simulink model "TEST_yuyao_all_BASIC_v2"  (R2023a)
settings: Solver=FixedStepDiscrete  StartTime=0.0  StopTime=inf  FixedStep=0.001  RelTol=1e-3  EnableMultiTasking=on
undefined symbols (not defined in the file or in its folder): IO397
libraries: slrealtimeseriallib x3, speedgoatlib_fpga_dio x2, speedgoatlib_fpga_analog_io x1, speedgoatlib_fpga x1
settings Model: Creator=Kalpana  LastModifiedBy=ysun
settings SolverCC: ConcurrentTasks=on  AlgebraicLoopSolver=TrustRegion  PositivePriorityOrder=on  InsertRTBMode=Never (minimum delay)
settings DataIOCC: SaveFormat=Array  SaveState=on  SignalLoggingName=logsOut
settings OptimizationCC: BlockReduction=off  BooleanDataType=off  OptimizeBlockIOStorage=off  BufferReuse=off  ReuseModelBlockBuffer=off  GlobalBufferReuse=off  ExpressionFolding=off  LocalBlockOutputs=off  InitFltsAndDblsToZero=on  OptimizeDataStoreBuffers=off  BusAssignmentInplaceUpdate=off
settings DebuggingCC: SaveWithParameterizedLinksMsg=none  UnderspecifiedInitializationDetection=Classic  MergeDetectMultiDrivingBlocksExec=none  CheckExecutionContextPreStartOutputMsg=on  SignalResolutionControl=TryResolveAllWithWarning  TasksWithSamePriorityMsg=none  UnconnectedInputMsg=warning  UnconnectedOutputMsg=warning  UnconnectedLineMsg=warning  SFUnexpectedBacktrackingDiag=warning  SFNoUnconditionalDefaultTransitionDiag=warning  SFExecutionAtInitializationDiag=none  ArithmeticOperatorsInVariantConditions=warning
settings HardwareCC: ProdBitPerLong=64  ProdLongLongMode=on  ProdHWDeviceType=Intel->x86-64 (Linux 64)
settings ModelReferenceCC: EnableRefExpFcnMdlSchedulingChecks=on  PropagateSignalLabelsOutOfModel=off
settings SFSimCC: SimUseLocalCustomCode=off  SimTargetLang=C++
settings RTWCC: Description=Simulink Real-Time  SystemTargetFile=slrealtime.tlc  TemplateMakefile=slrealtime_default_tmf  RTWUseLocalCustomCode=off  Toolchain=Simulink Real-Time Toolchain  BuildConfiguration=Faster Runs  CodeExecutionProfiling=on  TargetLang=C++  DLArmComputeVersion=19.05
settings CodeAppCC: StateflowObjectComments=on
settings SimulinkRealTimeTargetCC: MATLABClassNameForMDSCustomization=Simulink.SoftwareTarget.GRTCustomization  UseGCCFastMath=on
settings ConfigComp: CovMetricSettings=dw  CovSaveCumulativeToWorkspaceVar=on  CovSaveSingleToWorkspaceVar=on  CovExternalEMLEnable=off  CovSFcnEnable=off

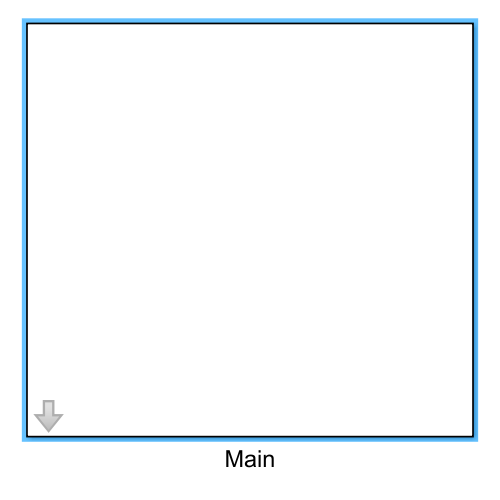
[thumbnail: Simulink's stored preview of the top-level diagram]
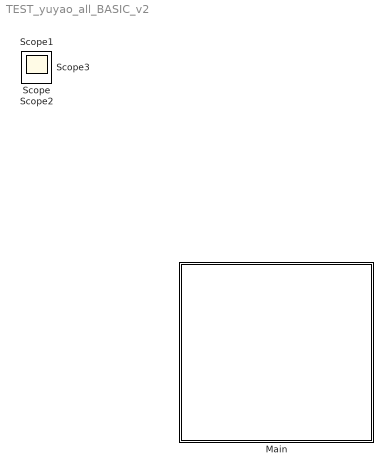
== system TEST_yuyao_all_BASIC_v2 ==
  Main : Subsystem  mask{iti_time=1, opp_time=500, deadtime=1000, water_time=1000, reaction_time=1000, target=10000}
      mask prompts: iti_time "inter trial interval duration (secs)"; opp_time "opportunity time (ms)"; deadtime "lick dead time (ms)"; water_time "water duration (ms)"; reaction_time "reaction_time(ms)"
      mask DialogControl win_parameters Prompt: Time Windows
  Scope{,1..3} (4 alike) : Scope

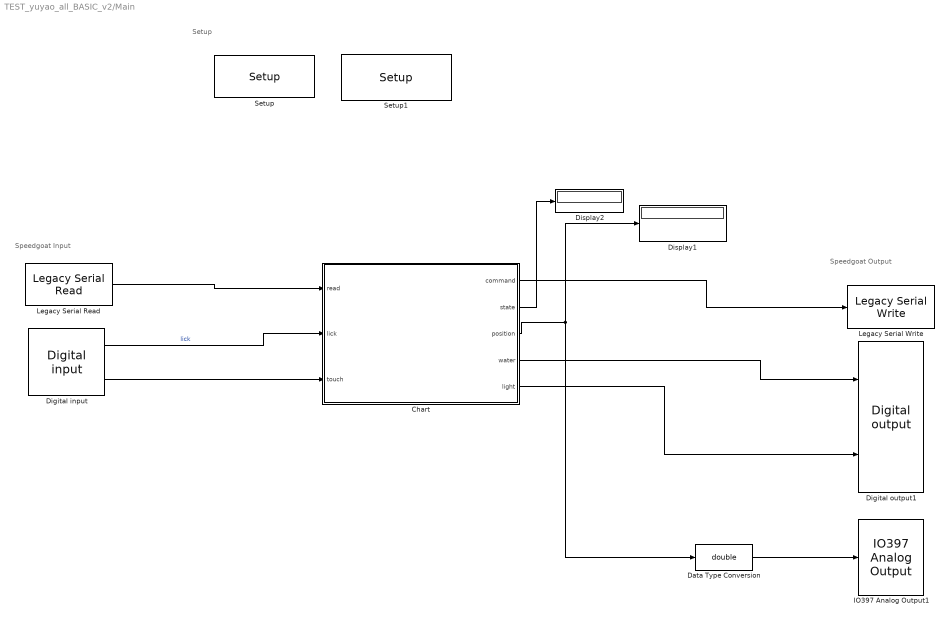
== system TEST_yuyao_all_BASIC_v2/Main ==
  note: Setup
  note: Speedgoat Input
  note: Speedgoat Output
  Chart : Stateflow chart  TreatAsAtomicUnit=on
      settings: PortSchema="{\"entries\":[{\"content\":{\"sides\":[{\"content\":{\"connectorIds\":[\"In1\",\"In2\",\"In3\"]},\"type\":\"ConnectorPlacement.EquallySpacedRectSide\",\"uuid\":\"c5c6425b-c61c-4cfd-8e89-a1433c662b1e\"},{\"content\":{\"connectorIds\":[\"Out1\",\"Out2\",\"Out3\",\"Out5\",\"Out4\"],\"side\":\"RIGHT\"},\"type\":\"ConnectorPlacement.EquallySpacedRectSide\",\"uuid\":\"e94e3558-7670-4901-8dc6-dcc10f25bbba\"},{\"content\":{\"side\":\"TOP\"},\"type\":\"ConnectorPlacement.EquallySpacedRectSide\",\"uuid\":\"e6d8a198-ffcd-48fe-900a-ac2ec65948b6\"}]},\"type\":\"ConnectorPlacement.EquallySpacedConnector\",\"uuid\":\"3d425b26-b95c-4585-983d-1dedea8cf8d0\"}],\"packageUris\":[\"http://schema.mathworks.com/mf0/Connector/R2020b\"],\"version\":\"1.0\"}"
  Data Type Conversion : DataTypeConversion  OutDataTypeStr=double  SaturateOnIntegerOverflow=off  RndMeth=Floor
  Digital input : speedgoatlib_fpga_dio/Digital input  id=1  chan=[1 5]  ts=0.01  pciSlot=-1  board=IO397-50k  vectorizeOutput=off
      settings: SourceProductName=Simulink Real-Time: Speedgoat I/O Blockset
  Digital output1 : speedgoatlib_fpga_dio/Digital output  id=1  chan=[2 6]  init=[0]  reset=[0]  vectorizeInput=off  ts=-1  pciSlot=-1  board=IO397-50k
      settings: SourceProductName=Simulink Real-Time: Speedgoat I/O Blockset
  Display1 : Display
  Display2 : Display
  IO397 Analog Output1 : speedgoatlib_fpga_analog_io/IO397 Analog Output  id=1  chan=[2]  initVal=0  resetVal=0  ts=0.01  pciSlot=-1  board=IO397-50k  span=+-5 V
      settings: SourceProductName=Simulink Real-Time: Speedgoat I/O Blockset
  Legacy Serial Read : slrealtimeseriallib/Mainboard/Legacy Serial Read  port=Legacy Serial Port 1  count=51  dtype=count+16 bit int  sampletime=.01
  Legacy Serial Write : slrealtimeseriallib/Mainboard/Legacy Serial Write  port=Legacy Serial Port 1  dtype=count+16 bit int  sampletime=.01
  Setup : slrealtimeseriallib/Mainboard/Setup  port=Legacy Serial Port 1  baud=115200  width=8  nstop=1  parity=None  ctsmode=off
  Setup1 : speedgoatlib_fpga/Setup/Setup  board=IO397-50k  id=1  device_id=1  frontIO=None  rearIO=None  bitstreamFile=speedgoat_IO397_50k_Comms.mat  rev=5.000000  timestamp_string=28/02/23 11:36:55  fpgaFreq=75 MHz  fpgaTick=13.33 ns  ProgSpiFlash=off  ProgBPIFlash=off  pciSlot=-1  PullRPort0=pull-up 3.3V  VioPort0=3.3V  PullRPort1=pull-up 3.3V  VioPort1=3.3V  PullRPort2=pull-up 3.3V  VioPort2=3.3V  PullRPort3=pull-up 3.3V  VioPort3=3.3V  PullRPort4=pull-up 3.3V  VioPort4=3.3V  PullRPort5=pull-up 3.3V  VioPort5=3.3V  PullRPort6=pull-up 3.3V  VioPort6=3.3V  diffLineTermination_rear1=on  diffLineTermination_rear2=on  diffLineTermination_rear3=on  diffLineTermination_rear4=on  diffLineTermination_rear5=on  diffLineTermination_rear6=on  diffLineTermination_rear7=on  diffLineTermination_rear8=on  PullRPort15=pull-up 3.3V  PullRPort31=pull-up 3.3V  PullRPort47=pull-up 3.3V  PullRPort63=pull-up 3.3V  diffLineTermination_1=on  diffLineTermination_2=on  diffLineTermination_3=on  diffLineTermination_4=on  diffLineTermination_5=on  diffLineTermination_6=on  diffLineTermination_7=on  diffLineTermination_8=on
      settings: SourceProductName=Simulink Real-Time: Speedgoat I/O Blockset
  wires:
  Data Type Conversion/1 -> IO397 Analog Output1/1
  Digital input/2 -> Chart/3(touch)
  Chart/5(water) -> Digital output1/1
  Legacy Serial Read/1 -> Chart/1(read)
  Chart/2(state) -> Display2/1
  Chart/1(command) -> Legacy Serial Write/1
  Chart/3(position) -> Data Type Conversion/1, Display1/1
  Chart/4(light) -> Digital output1/2
  Digital input/1 -> Chart/2(lick)  "lick"

== stateflow chart TEST_yuyao_all_BASIC_v2/Main/Chart ==
  state Motor
    entry:
    state = 0;
    during:
    on setenable_1: command =  int16([0x0014 0x0090 0x0002 0x0068 0x0004 0x0001 0x0040 0x0060 0x0000 0x0006 0x0000 0x0000 0x0000 0x0022 0x0099]);
    on setenable_2: command =  int16([0x0014 0x0090 0x0002 0x0068 0x0004 0x0001 0x0040 0x0060 0x0000 0x000F 0x0000 0x0000 0x0000 0x00B3 0x0007]);
    on clearerror_1: command =  int16([0x0014 0x0090 0x0002 0x0068 0x0004 0x0001 0x0003 0x0010 0x0000 0x0000 0x0000 0x0000 0x0000 0x00A1 0x0008]);
    on clearerror_2: command =  int16([0x0014 0x0090 0x0002 0x0068 0x0004 0x0001 0x0040 0x0060 0x0000 0x0000 0x0000 0x0000 0x0000 0x0082 0x002B]);
    on clearerror_3: command =  int16([0x0014 0x0090 0x0002 0x0068 0x0004 0x0001 0x0040 0x0060 0x0000 0x0080 0x0000 0x0000 0x0000 0x00D8 0x0010]);
    on getposition: command =  int16([0x0010 0x0090 0x0002 0x0060 0x0002 0x0001 0x0064 0x0060 0x0000 0x0029 0x005A 0x0000 0x0000 0x0000 0x0000 ]);
    on SetoperationMode: command = int16([0x0014 0x0090 0x0002 0x0068 0x0004 0x0001 0x0060 0x0060 0x0000 0x0001 0x0000 0x0000 0x0000 0x00DA 0x0067]);
    on getmovementstate: command = int16([0x0010 0x0090 0x0002 0x0060 0x0002 0x0001 0x0041 0x0060 0x0000 0x0022 0x00D1 0x0000 0x0000 0x0000 0x0000]);
    on Torque_mode: command = int16([0x0014 0x0090 0x0002 0x0068 0x0004 0x0001 0x0060 0x0060 0x0000 0x000A 0x0000 0x0000 0x0000 0x002B 0x0097]);
    on Torque: command = int16([0x0014 0x0090 0x0002 0x0068 0x0004 0x0001 0x0071 0x0060 0x0000 0x0030 0x00F8 0x00FF 0x00FF 0x00A9 0x00E8]);
    on setdisable:command = int16([0x0014 0x0090 0x0002 0x0068 0x0004 0x0001 0x0040 0x0060 0x0000 0x0000 0x0000 0x0000 0x0000 0x0082 0x002B]);
    on CSP_mode: command = int16([0x0014 0x0090 0x0002 0x0068 0x0004 0x0001 0x0060 0x0060 0x0000 0x0008 0x0000 0x0000 0x0000 0x004B 0x00F9]);
    on moveto0: command = int16([0x0014 0x0090 0x0002 0x0068 0x0004 0x0001 0x007A 0x0060 0x0000 0x0000 0x0000 0x0000 0x0000 0x0022 0x00FC]);
    state Getposition
      entry:
      getposition
      during:
      position = extractAndMerge(read);
      state State
        en:
        state = 2;
      state Pull
        en:
        state = 3;
      (default) -> State
      State -> Pull : [any(position >= target)]
    state ITI
    state ProgStart
      state SETENABLE_2
        entry:
        setenable_2
      state CLEARERROR
        entry:
        clearerror_1
      state SETENABLE
        entry:
        setenable_1
      state exit
        entry:
        state = 1;
      state CLEARERROR2
        entry:
        clearerror_2
      state CLEARERROR3
        entry:
        clearerror_3
      (default) -> Motor.ProgStart.SETENABLE
      Motor.ProgStart.SETENABLE_2 -> CLEARERROR : [after(10,msec)]
      Motor.ProgStart.SETENABLE -> Motor.ProgStart.SETENABLE_2 : [after(10,msec)]
      CLEARERROR -> CLEARERROR2 : [after(10,msec)]
      CLEARERROR2 -> CLEARERROR3 : [after(10,msec)]
      CLEARERROR3 -> exit : [after(10,msec)]
    state wait
    state lightOFF
      entry:
      light=0;
    state LightON
      entry:
      light=1;
    state WaterON
      entry:
      water = 1;
      ex:
      state = 6;
    state WaterOFF
      entry:
      water = 0;
    state Lickingtime
    state Getposition2
      entry:
      getposition
      during:
      position = extractAndMerge(read);
      state Position1
      state Position2
        en:
        state = 8;
      state Position3
        en:
        state =9;
      (default) -> Position1
      Position1 -> Position2 [order 1] : [any(position <= 500)]
      Position1 -> Position3 [order 4] : [any(position < -500)]
      Position1 -> Position3 [order 3] : [any(position > 500)]
      Position1 -> Position2 [order 2] : [any(position >= -500)]
    state ToMidpoint
      state SETENABLE_2
        entry:
        setenable_2
      state SETENABLE
        entry:
        setenable_1
      state CSP
        entry:
        CSP_mode
      state Torque
        en:
        Torque
      state MOVE
        entry:
        moveto0
      state MOVE1
        entry:
        state = 7;
      (default) -> Motor.ToMidpoint.SETENABLE
      Motor.ToMidpoint.SETENABLE -> Motor.ToMidpoint.SETENABLE_2 : [after(10,msec)]
      Motor.ToMidpoint.SETENABLE_2 -> CSP : [after(10,msec)]
      CSP -> Torque : [after(10,msec)]
      Torque -> MOVE : [after(10,msec)]
      MOVE -> MOVE1 : [after(10,msec)]
    ProgStart -> ITI : [state == 1]
    ITI -> Getposition : [after(iti_time,sec)]
    Getposition -> wait [order 1] : [state == 3]
    Getposition -> LightON [order 2] : [~touch|after(10,sec)]{state = 4;}
    (default) -> ProgStart
    Getposition2 -> LightON [order 1] : [state ==9]
    lightOFF -> ProgStart
    wait -> WaterON : [after(0.2,sec)]
    LightON -> ToMidpoint
    Getposition2 -> lightOFF [order 2] : [state ==8]
    WaterOFF -> Lickingtime : [after(reaction_time,msec)|lick]
    Lickingtime -> ToMidpoint [order 1] : [after(deadtime, msec)]
    WaterON -> WaterOFF : [after(water_time, msec)]
    Lickingtime -> Lickingtime [order 2] : [lick]
    ToMidpoint -> Getposition2 : [state ==7]
  data: position function_input; motorPosition function_output; command output; state output double; read input; targetpushposition local; targetpullposition local; position output; status local; light output; lick input; water output; touch input; deadtime parameter; iti_time parameter; reaction_time parameter; water_time parameter; target parameter
  events: setenable_1 local FUNCTION_CALL_EVENT; setenable_2 local FUNCTION_CALL_EVENT; clearerror_2 local FUNCTION_CALL_EVENT; clearerror_3 local FUNCTION_CALL_EVENT; clearerror_1 local FUNCTION_CALL_EVENT; getposition local FUNCTION_CALL_EVENT; SetoperationMode local FUNCTION_CALL_EVENT; Setpositionprofile_speed_1 local FUNCTION_CALL_EVENT; Setpositionprofile_acceleration_1 local FUNCTION_CALL_EVENT; Setpositionprofile_deceleration_1 local FUNCTION_CALL_EVENT; Movetoposition_settarget_1 local FUNCTION_CALL_EVENT; Movetoposition_gotarget_1 local FUNCTION_CALL_EVENT; Movetoposition_gotarget_2 local FUNCTION_CALL_EVENT; Movetoposition_settarget_2 local FUNCTION_CALL_EVENT; Setpositionprofile_acceleration_2 local FUNCTION_CALL_EVENT; Setpositionprofile_deceleration_2 local FUNCTION_CALL_EVENT; Setpositionprofile_speed_2 local FUNCTION_CALL_EVENT; Movetoposition_gotarget2 local FUNCTION_CALL_EVENT; getmovementstate local FUNCTION_CALL_EVENT; Torque local FUNCTION_CALL_EVENT; setdisable local FUNCTION_CALL_EVENT; Torque_mode local FUNCTION_CALL_EVENT; moveto0 local FUNCTION_CALL_EVENT; CSP_mode local FUNCTION_CALL_EVENT
  function motorPosition = extractAndMerge(position):
    | function motorPosition = extractAndMerge(position)
    | 
    |      startByte = 10;
    |      endByte = 13;
    |      extractedData = position(startByte:endByte);
    |      mergedValue = int32(0);
    |      for i = length(extractedData):-1:1
    |          mergedValue = bitor(bitshift(mergedValue,8), int32(extractedData(i)));
    |      end
    |      motorPosition = mergedValue;
    |      % motorPosition = typecast(mergedValue,'int32');
    | 
    | end
